simulink library "ddm"  (R2021b)
settings: Solver=VariableStepAuto  StartTime=0.0  StopTime=10.0  RelTol=1e-3
undefined symbols (not defined in the file or in its folder): ENUM_ADASACCSTA_ERROR, ENUM_ADASACCSTA_OFF, ENUM_ADASACCSTA_STANDBY, ENUM_ADASISASTA_OFF, ENUM_ALLOWMOV_ALLOWREADY, ENUM_APS, ENUM_BRKSTA_ERROR, ENUM_BRKSTA_OFF, ENUM_BRKSTA_ON, ENUM_BRKSW_INVALID, ENUM_BRKSW_OFF, ENUM_BRKSW_ON, ENUM_CHGPREACTERRSTA_OBCPRE, ENUM_DCDCFAULTSTA_ANYFAULTLV1, ENUM_DCDCFAULTSTA_ANYFAULTLV2, ENUM_DRIVETRAIN_AWD, ENUM_DRIVETRAIN_FWD, ENUM_DRIVETRAIN_RWD, ENUM_DRSEATSTA_INVALID, ENUM_EDUDRTSTA_NORMAL, ENUM_EPBSTA_APPLIED, ENUM_EPBSTA_RELEASED, ENUM_HVBATTREADYPRE_READY, ENUM_MCUWARN_LV0, ENUM_MCUWARN_LV1, ENUM_MCUWARN_LV2, ENUM_MCUWARN_LV3, ENUM_MCUWARN_NOERROR, ENUM_OBCFAULTSTA_ANYFAULT, ENUM_PAS_R2F2, ENUM_PDFAULT_BATTPDFAIL, ENUM_PDFAULT_DCDCDISABLE, ENUM_PDFAULT_MCUDISABLE, ENUM_PDFAULT_MCUDISCHRG, ENUM_POWERSTA_OFF, ENUM_POWERSTA_ON, ENUM_POWERSTA_READY, ENUM_POWERSTA_STANDBY, ENUM_PRESSINDI_LOW, ENUM_PUFAULT_BATTUPFAIL, ENUM_PUFAULT_DCDCENABLEFAIL, ENUM_PUFAULT_PRECHRGCHKFAIL, ENUM_PUFAULT_SAFETYCHKFAIL, ENUM_PUSTATE_COMPLETED, ENUM_PWRSTASW_OFF, ENUM_PWRSTASW_OFFA, ENUM_PWRSTASW_OFFCHVCHRG, ENUM_PWRSTASW_OFFCLVCHRG, ENUM_PWRSTASW_ON, ENUM_PWRSTASW_ONHVCHRG, ENUM_PWRSTASW_READY, ENUM_PWRSTASW_STANDBY, ENUM_RANGESTA_12IN, ENUM_SHIFTCOMMAND_D, ENUM_SHIFTCOMMAND_N, ENUM_SHIFTCOMMAND_P, ENUM_SHIFTCOMMAND_R, ENUM_VEHMALFUNLV_2ND, ENUM_VEHMALFUNLV_3RD, ENUM_VEHMALFUNLV_4TH ... (+835)
libraries: hcu_lib x750, $bdroot x12, simulink x5
(part 20 of 28)

== system ddm/DDM/DDM/PMM/SW failure/Hood switch failure ==
  note: Diagnostics and Fault Handling
  note: Fail Safe During Detection
  note: Fail Safe After Decision
  note: Release Condition After Decision
  note: Release Condition During Detection
  note: Test Pass Criteria
  note: Test Detection Criteria
  task_time_s : Inport
  VPMM_PowerSta_enum : Inport  Port=2
  VPMM_PwrStaSW_enum : Inport  Port=3
  VINP_HoodSW : Inport  Port=4
  DTC_clear_request : Inport  Port=5
  Constant{10,18,53,55} (4 alike) : Constant  Value=FALSE
  Constant11 : Constant  Value=KDDM_HoodSWPassTO_s
  Constant15 : Constant  Value=KDDM_HoodSWPassTO_s
  Constant16 : Constant  Value=KDDM_HoodSWDetTO_s
  Constant17 : Constant  Value=KDDM_HoodSW_s
  Constant19 : Constant  Value=ENUM_PWRSTASW_OFF
  Constant21 : Constant  Value=ZERO_INT
  Constant22 : Constant  Value=ENUM_PWRSTASW_OFF
  Constant{23,42,52,54} (4 alike) : Constant  Value=TRUE
  Constant24 : Constant  Value=KDDM_HoodSWPassTO_s
  Constant25 : Constant  Value=KDDM_HoodSWDTC_cnt
  Constant26 : Constant  Value=ONE_INT
  Constant32 : Constant  Value=ZERO_FLOAT
  Constant45 : Constant  Value=ENUM_POWERSTA_OFF
  Constant56 : Constant  Value=KDDM_HoodSWPassSW_flg
  Constant57 : Constant  Value=KDDM_HoodSWCFSSW_flg
  Constant58 : Constant  Value=KDDM_HoodSWDFSSW_flg
  Constant59 : Constant  Value=KDDM_HoodSWDetSW_flg
  Constant60 : Constant  Value=KDDM_HoodSWDTC_cnt
  DTC_Couter1 : hcu_lib/Basic_Blocks/DTC_Couter
  DTC_Info : hcu_lib/Basic_Blocks/DTC_Info
  Data Type Conversion12 : DataTypeConversion  OutDataTypeStr=boolean
  Data Type Conversion14 : DataTypeConversion  OutDataTypeStr=boolean
  Data Type Conversion4 : DataTypeConversion  OutDataTypeStr=uint8
  Data Type Conversion7 : DataTypeConversion
  Equal1 : RelationalOperator  Operator=~=  OutDataTypeStr=boolean  RndMeth=Simplest
  Equal3 : RelationalOperator  Operator=~=  OutDataTypeStr=boolean  RndMeth=Simplest
  Equal4 : RelationalOperator  Operator=~=  OutDataTypeStr=boolean  RndMeth=Simplest
  Equal5 : RelationalOperator  OutDataTypeStr=boolean  RndMeth=Simplest
  Equal8 : RelationalOperator  Operator===  OutDataTypeStr=boolean  RndMeth=Simplest
  Logical Operator{2,4..5,7} (4 alike) : Logic  Operator=NOT  AllPortsSameDT=off  OutDataTypeStr=boolean
  Logical Operator27 : Logic  Operator=OR  AllPortsSameDT=off  OutDataTypeStr=boolean
  Logical Operator{6,28..30} (4 alike) : Logic  AllPortsSameDT=off  OutDataTypeStr=boolean
  Logical Operator3 : Logic  Operator=OR  AllPortsSameDT=off  OutDataTypeStr=boolean
  Logical Operator31 : Logic  Inputs=3  AllPortsSameDT=off  OutDataTypeStr=boolean
  Logical Operator32 : Logic  Operator=OR  Inputs=3  AllPortsSameDT=off  OutDataTypeStr=boolean
  Logical Operator33 : Logic  Operator=OR  Inputs=3  AllPortsSameDT=off  OutDataTypeStr=boolean
  Relational Operator4 : RelationalOperator  Operator=<=  OutDataTypeStr=boolean  RndMeth=Simplest
  Relational Operator5 : RelationalOperator  Operator=>  OutDataTypeStr=boolean  RndMeth=Simplest
  Relay1 : Relay  OnSwitchValue=ONE_INT  OffSwitchValue=ZERO_INT
  SR_Latch1 : hcu_lib/Basic_Blocks/SR_Latch
  SR_Latch2 : hcu_lib/Basic_Blocks/SR_Latch
  SR_Latch3 : $bdroot/DDM/DDM/PMM/SW failure/Driver seat switch failure/SR_Latch3
  SR_Latch5 : hcu_lib/Basic_Blocks/SR_Latch
  Subsystem : $bdroot/DDM/DDM/PMM/SW failure/Driver seat switch failure/Subsystem  SystemSampleTime=-1  VariantActivationTime=update diagram  Latency=0  AutoFrameSizeCalculation=off
      link override Constant15: Value=KDDM_HoodSW_s
  Switch{5,10..11,14..16} (6 alike) : Switch  Criteria=u2 ~= 0
  Test Detection Criteria2 : hcu_lib/Basic_Blocks/Test Detection Criteria
  Timer : hcu_lib/Basic_Blocks/Test Detection Criteria/Timer
  Timer1 : hcu_lib/Basic_Blocks/Timer
  Unit Delay : UnitDelay  SampleTime=-1  HasFrameUpgradeWarning=on
  Unit Delay9 : UnitDelay  SampleTime=-1  HasFrameUpgradeWarning=on
  VDDM_HoodSWDTC_raw32 : Outport
  VDDM_VCUHoodSWSta_flg : Outport  Port=2
  wires:
  Logical Operator31/1 -> DTC_Couter1/1
  [DTC_clear_request] -> Logical Operator3/2
  SR_Latch5/1 -> Logical Operator30/1
  Logical Operator3/1 -> SR_Latch5/2
  Logical Operator28/1 -> [VDDM_HoodSWDFS_flg]
  Logical Operator2/1 -> Logical Operator31/3
  [VDDM_HoodSWPass_flg] -> Logical Operator33/1
  DTC_Couter1/2 -> Data Type Conversion4/1
  [DTC_clear_request] -> Logical Operator2/1
  [DTC_clear_request] -> Logical Operator32/3
  [DTC_clear_request] -> Logical Operator33/3
  Logical Operator33/1 -> Logical Operator29/1
  Data Type Conversion4/1 -> [VDDM_HoodSWDTC_cnt]  "VDDM_HoodSWDTC_cnt"
  Relay1/1 -> SR_Latch2/1
  [VDDM_HoodSWCFSRls_flg] -> Logical Operator3/1
  [VDDM_HoodSWDTC_cnt] -> Relay1/1
  [VDDM_HoodSWDet_flg] -> Logical Operator31/1
  Constant57/1 -> Logical Operator30/2
  Logical Operator32/1 -> SR_Latch2/2
  Logical Operator29/1 -> DTC_Couter1/2
  Logical Operator30/1 -> [VDDM_HoodSWCFS_flg]  "VDDM_HoodSWCFS_flg"
  Constant58/1 -> Logical Operator28/1
  Constant59/1 -> Logical Operator31/2
  Constant60/1 -> DTC_Couter1/3
  Constant56/1 -> Logical Operator29/2
  [VDDM_HoodSWDFSRls_flg] -> Logical Operator32/1
  DTC_Couter1/1 -> SR_Latch5/1
  [VDDM_HoodSWCFSRls_flg] -> Logical Operator33/2
  [VDDM_HoodSWCFS_flg] -> Logical Operator32/2
  SR_Latch2/1 -> Logical Operator28/2
  [DTC_clear_request] -> DTC_Info/4
  [VDDM_HoodSWDet_flg] -> DTC_Info/1
  [VDDM_HoodSWCFS_flg] -> DTC_Info/3
  [VDDM_HoodSWPass_flg] -> DTC_Info/2
  DTC_Info/1 -> VDDM_HoodSWDTC_raw32/1  "VDDM_HoodSWDTC_raw32"
  Constant10/1 -> Switch11/3
  VPMM_PwrStaSW_enum/1 -> [VPMM_PwrStaSW_enum]
  VPMM_PowerSta_enum/1 -> [VPMM_PowerSta_enum]
  DTC_clear_request/1 -> [DTC_clear_request]
  VINP_HoodSW/1 -> [VINP_HoodSWGPIO_flg]
  task_time_s/1 -> [task_time_s]
  [VDDM_HoodSWCFS_flg] -> Switch11/2
  Constant42/1 -> Switch11/1
  Switch11/1 -> [VDDM_VCUHoodSWSta_flg]  "VDDM_VCUHoodSWSta_flg"
  Logical Operator27/1 -> Switch15/2
  Constant52/1 -> Switch16/1
  Equal8/1 -> Logical Operator27/1
  [VDDM_HoodSWPass_flg] -> Switch16/2
  Constant53/1 -> Switch16/3
  Constant45/1 -> Equal8/2
  Constant55/1 -> Switch15/3
  Switch15/1 -> [VDDM_HoodSWCFSRls_flg]  "VDDM_HoodSWCFSRls_flg"
  Switch16/1 -> [VDDM_HoodSWDFSRls_flg]
  [DTC_clear_request] -> Logical Operator27/2
  Constant54/1 -> Switch15/1
  [VPMM_PowerSta_enum] -> Equal8/1
  [VDDM_VCUHoodSWSta_flg] -> VDDM_VCUHoodSWSta_flg/1
  [VDDM_HoodSWChange_flg] -> SR_Latch1/2
  Logical Operator7/1 -> Timer1/1
  Data Type Conversion7/1 -> Test Detection Criteria2/4
  Subsystem/1 -> Logical Operator6/1
  Equal4/1 -> [VDDM_HoodSWChange_flg]
  Test Detection Criteria2/1 -> [VDDM_HoodSWDet_flg]  "VDDM_HoodSWDet_flg"
  Switch10/1 -> Logical Operator7/1, Timer1/2
  Constant32/1 -> Relational Operator5/2
  [VPMM_PwrStaSW_enum] -> Equal1/1
  [VDDM_xxx_flg] -> SR_Latch3/2
  Relational Operator4/1 -> Logical Operator6/2
  Constant26/1 -> SR_Latch1/1
  [task_time_s] -> Timer1/3
  Constant21/1 -> Switch14/3
  [task_time_s] -> Timer/3
  Constant22/1 -> Equal1/2
  Data Type Conversion14/1 -> Equal4/1
  SR_Latch1/1 -> Logical Operator5/1, Logical Operator4/1, Timer/1
  Switch5/1 -> Data Type Conversion12/1
  Constant23/1 -> Switch10/3
  Data Type Conversion12/1 -> Test Detection Criteria2/1
  Logical Operator6/1 -> [HoodSWFault_flg], Switch14/1
  Constant17/1 -> Relational Operator4/2
  Constant11/1 -> Timer/4
  Unit Delay/1 -> Subsystem/1
  Logical Operator4/1 -> Timer/2
  Constant25/1 -> Test Detection Criteria2/3
  [task_time_s] -> Test Detection Criteria2/2
  Constant18/1 -> Switch5/1
  Relational Operator5/1 -> Unit Delay9/1, Equal4/2
  [DTC_clear_request] -> Switch5/2
  Logical Operator5/1 -> Subsystem/Trigger
  Constant16/1 -> Data Type Conversion7/1
  Constant24/1 -> Equal5/2
  Timer1/1 -> Equal5/1
  Timer/1 -> Relational Operator4/1, Unit Delay/1
  Constant15/1 -> Timer1/4
  Unit Delay9/1 -> Data Type Conversion14/1
  Equal3/1 -> Switch10/2
  Equal5/1 -> SR_Latch3/1
  Equal1/1 -> Switch14/2
  Switch14/1 -> [VDDM_xxx_flg], Switch5/3
  [HoodSWFault_flg] -> Switch10/1
  [VINP_HoodSWGPIO_flg] -> Relational Operator5/1
  [VPMM_PwrStaSW_enum] -> Equal3/1
  SR_Latch3/1 -> [VDDM_HoodSWPass_flg]  "VDDM_HoodSWPass_flg"
  Constant19/1 -> Equal3/2

== system ddm/DDM/DDM/PMM/SW failure/RL Door switch failure ==
  note: Diagnostics and Fault Handling
  note: Release Condition During Detection
  note: Release Condition After Decision
  note: Fail Safe After Decision
  note: Fail Safe During Detection
  note: Test Pass Criteria
  note: Test Detection Criteria
  task_time_s : Inport
  VPMM_PowerSta_enum : Inport  Port=2
  VPMM_PwrStaSW_enum : Inport  Port=3
  VINP_RLAJARSW : Inport  Port=4
  DTC_clear_request : Inport  Port=5
  Constant{10,18,53,55} (4 alike) : Constant  Value=FALSE
  Constant11 : Constant  Value=KDDM_RLDoorSWPassTO_s
  Constant15 : Constant  Value=KDDM_RLDoorSWPassTO_s
  Constant16 : Constant  Value=KDDM_RLDoorSWDetTO_s
  Constant17 : Constant  Value=KDDM_RLDoorSW_s
  Constant19 : Constant  Value=ENUM_PWRSTASW_OFF
  Constant21 : Constant  Value=ZERO_INT
  Constant22 : Constant  Value=ENUM_PWRSTASW_OFF
  Constant{23,42,52,54} (4 alike) : Constant  Value=TRUE
  Constant24 : Constant  Value=KDDM_RLDoorSWPassTO_s
  Constant25 : Constant  Value=KDDM_RLDoorSWDTC_cnt
  Constant26 : Constant  Value=ONE_INT
  Constant32 : Constant  Value=ZERO_FLOAT
  Constant45 : Constant  Value=ENUM_POWERSTA_OFF
  Constant56 : Constant  Value=KDDM_RLDoorSWPassSW_flg
  Constant57 : Constant  Value=KDDM_RLDoorSWCFSSW_flg
  Constant58 : Constant  Value=KDDM_RLDoorSWDFSSW_flg
  Constant59 : Constant  Value=KDDM_RLDoorSWDetSW_flg
  Constant60 : Constant  Value=KDDM_RLDoorSWDTC_cnt
  DTC_Couter1 : hcu_lib/Basic_Blocks/DTC_Couter
  DTC_Info : hcu_lib/Basic_Blocks/DTC_Info
  Data Type Conversion10 : DataTypeConversion  OutDataTypeStr=boolean
  Data Type Conversion13 : DataTypeConversion
  Data Type Conversion14 : DataTypeConversion  OutDataTypeStr=boolean
  Data Type Conversion4 : DataTypeConversion  OutDataTypeStr=uint8
  Equal1 : RelationalOperator  Operator=~=  OutDataTypeStr=boolean  RndMeth=Simplest
  Equal3 : RelationalOperator  Operator=~=  OutDataTypeStr=boolean  RndMeth=Simplest
  Equal4 : RelationalOperator  Operator=~=  OutDataTypeStr=boolean  RndMeth=Simplest
  Equal5 : RelationalOperator  OutDataTypeStr=boolean  RndMeth=Simplest
  Equal8 : RelationalOperator  Operator===  OutDataTypeStr=boolean  RndMeth=Simplest
  Logical Operator{2,4..5,7} (4 alike) : Logic  Operator=NOT  AllPortsSameDT=off  OutDataTypeStr=boolean
  Logical Operator27 : Logic  Operator=OR  AllPortsSameDT=off  OutDataTypeStr=boolean
  Logical Operator{6,28..30} (4 alike) : Logic  AllPortsSameDT=off  OutDataTypeStr=boolean
  Logical Operator3 : Logic  Operator=OR  AllPortsSameDT=off  OutDataTypeStr=boolean
  Logical Operator31 : Logic  Inputs=3  AllPortsSameDT=off  OutDataTypeStr=boolean
  Logical Operator32 : Logic  Operator=OR  Inputs=3  AllPortsSameDT=off  OutDataTypeStr=boolean
  Logical Operator33 : Logic  Operator=OR  Inputs=3  AllPortsSameDT=off  OutDataTypeStr=boolean
  Relational Operator4 : RelationalOperator  Operator=<=  OutDataTypeStr=boolean  RndMeth=Simplest
  Relational Operator5 : RelationalOperator  Operator=>  OutDataTypeStr=boolean  RndMeth=Simplest
  Relay1 : Relay  OnSwitchValue=ONE_INT  OffSwitchValue=ZERO_INT
  SR_Latch1 : hcu_lib/Basic_Blocks/SR_Latch
  SR_Latch2 : hcu_lib/Basic_Blocks/SR_Latch
  SR_Latch3 : $bdroot/DDM/DDM/PMM/SW failure/Driver seat switch failure/SR_Latch3
  SR_Latch5 : hcu_lib/Basic_Blocks/SR_Latch
  Subsystem : $bdroot/DDM/DDM/PMM/SW failure/Driver seat switch failure/Subsystem  SystemSampleTime=-1  VariantActivationTime=update diagram  Latency=0  AutoFrameSizeCalculation=off
      link override Constant15: Value=KDDM_RLDoorSW_s
  Switch{5,10..11,14..16} (6 alike) : Switch  Criteria=u2 ~= 0
  Test Detection Criteria2 : hcu_lib/Basic_Blocks/Test Detection Criteria
  Timer : hcu_lib/Basic_Blocks/Test Detection Criteria/Timer
  Timer1 : hcu_lib/Basic_Blocks/Timer
  Unit Delay : UnitDelay  SampleTime=-1  HasFrameUpgradeWarning=on
  Unit Delay9 : UnitDelay  SampleTime=-1  HasFrameUpgradeWarning=on
  VDDM_RLDoorSWDTC_raw32 : Outport
  VDDM_VCURLDoorSta_flg : Outport  Port=2
  wires:
  Data Type Conversion4/1 -> [VDDM_RLDoorSWDTC_cnt]
  [VDDM_RLDoorSWPass_flg] -> Logical Operator33/1
  DTC_Couter1/1 -> SR_Latch5/1
  SR_Latch2/1 -> Logical Operator28/2
  [DTC_clear_request] -> Logical Operator32/3
  [VDDM_RLDoorSWCFSRls_flg] -> Logical Operator3/1
  Logical Operator2/1 -> Logical Operator31/3
  [VDDM_RLDoorSWCFSRls_flg] -> Logical Operator33/2
  Logical Operator30/1 -> [VDDM_RLDoorSWCFS_flg]  "VDDM_RLDoorSWCFS_flg"
  Constant56/1 -> Logical Operator29/2
  Constant57/1 -> Logical Operator30/2
  Constant59/1 -> Logical Operator31/2
  Logical Operator29/1 -> DTC_Couter1/2
  DTC_Couter1/2 -> Data Type Conversion4/1
  SR_Latch5/1 -> Logical Operator30/1
  [VDDM_RLDoorSWDFSRls_flg] -> Logical Operator32/1
  [VDDM_RLDoorSWDTC_cnt] -> Relay1/1
  [VDDM_RLDoorSWDet_flg] -> Logical Operator31/1
  Logical Operator3/1 -> SR_Latch5/2
  Relay1/1 -> SR_Latch2/1
  Constant58/1 -> Logical Operator28/1
  Logical Operator32/1 -> SR_Latch2/2
  Logical Operator28/1 -> [VDDM_RLDoorSWDFS_flg]
  [DTC_clear_request] -> Logical Operator3/2
  [DTC_clear_request] -> Logical Operator33/3
  [VDDM_RLDoorSWCFS_flg] -> Logical Operator32/2
  Logical Operator33/1 -> Logical Operator29/1
  Logical Operator31/1 -> DTC_Couter1/1
  [DTC_clear_request] -> Logical Operator2/1
  Constant60/1 -> DTC_Couter1/3
  [DTC_clear_request] -> DTC_Info/4
  [VDDM_RLDoorSWDet_flg] -> DTC_Info/1
  DTC_Info/1 -> VDDM_RLDoorSWDTC_raw32/1  "VDDM_RLDoorSWDTC_raw32"
  [VDDM_RLDoorSWCFS_flg] -> DTC_Info/3
  [VDDM_RLDoorSWPass_flg] -> DTC_Info/2
  Constant10/1 -> Switch11/3
  VPMM_PowerSta_enum/1 -> [VPMM_PowerSta_enum]
  VPMM_PwrStaSW_enum/1 -> [VPMM_PwrStaSW_enum]
  [VDDM_VCURLDoorSta_flg] -> VDDM_VCURLDoorSta_flg/1
  [VPMM_PowerSta_enum] -> Equal8/1
  Constant54/1 -> Switch15/1
  [DTC_clear_request] -> Logical Operator27/2
  Switch16/1 -> [VDDM_RLDoorSWDFSRls_flg]
  Switch15/1 -> [VDDM_RLDoorSWCFSRls_flg]  "VDDM_RLDoorSWCFSRls_flg"
  Constant55/1 -> Switch15/3
  Constant45/1 -> Equal8/2
  Constant53/1 -> Switch16/3
  [VDDM_RLDoorSWPass_flg] -> Switch16/2
  Equal8/1 -> Logical Operator27/1
  Constant52/1 -> Switch16/1
  Logical Operator27/1 -> Switch15/2
  Switch11/1 -> [VDDM_VCURLDoorSta_flg]  "VDDM_VCURLDoorSta_flg"
  Constant42/1 -> Switch11/1
  [VDDM_RLDoorSWCFS_flg] -> Switch11/2
  task_time_s/1 -> [task_time_s]
  VINP_RLAJARSW/1 -> [VINP_RL_AJAR_SW]
  DTC_clear_request/1 -> [DTC_clear_request]
  Data Type Conversion14/1 -> Equal4/1
  Constant23/1 -> Switch10/3
  [task_time_s] -> Timer1/3
  Constant22/1 -> Equal1/2
  [task_time_s] -> Timer/3
  Constant21/1 -> Switch14/3
  Constant26/1 -> SR_Latch1/1
  [task_time_s] -> Test Detection Criteria2/2
  [RLDoorSWFault_flg] -> Switch10/1
  Logical Operator7/1 -> Timer1/1
  Timer1/1 -> Equal5/1
  Logical Operator4/1 -> Timer/2
  Data Type Conversion10/1 -> Test Detection Criteria2/1
  Data Type Conversion13/1 -> Test Detection Criteria2/4
  [VDDM_xxx_flg] -> SR_Latch3/2
  Unit Delay/1 -> Subsystem/1
  Constant25/1 -> Test Detection Criteria2/3
  Constant24/1 -> Equal5/2
  Subsystem/1 -> Logical Operator6/1
  Equal1/1 -> Switch14/2
  [DTC_clear_request] -> Switch5/2
  Constant16/1 -> Data Type Conversion13/1
  [VPMM_PwrStaSW_enum] -> Equal3/1
  Constant11/1 -> Timer/4
  Switch5/1 -> Data Type Conversion10/1
  Switch14/1 -> [VDDM_xxx_flg], Switch5/3
  SR_Latch1/1 -> Logical Operator5/1, Logical Operator4/1, Timer/1
  Relational Operator4/1 -> Logical Operator6/2
  Constant18/1 -> Switch5/1
  SR_Latch3/1 -> [VDDM_RLDoorSWPass_flg]  "VDDM_RLDoorSWPass_flg"
  Equal5/1 -> SR_Latch3/1
  Constant17/1 -> Relational Operator4/2
  Constant15/1 -> Timer1/4
  Equal3/1 -> Switch10/2
  Logical Operator6/1 -> [RLDoorSWFault_flg], Switch14/1
  [VPMM_PwrStaSW_enum] -> Equal1/1
  Logical Operator5/1 -> Subsystem/Trigger
  [VDDM_RLDoorSWChange_flg] -> SR_Latch1/2
  Relational Operator5/1 -> Unit Delay9/1, Equal4/2
  Unit Delay9/1 -> Data Type Conversion14/1
  Timer/1 -> Relational Operator4/1, Unit Delay/1
  [VINP_RL_AJAR_SW] -> Relational Operator5/1
  Constant19/1 -> Equal3/2
  Equal4/1 -> [VDDM_RLDoorSWChange_flg]
  Switch10/1 -> Logical Operator7/1, Timer1/2
  Constant32/1 -> Relational Operator5/2
  Test Detection Criteria2/1 -> [VDDM_RLDoorSWDet_flg]  "VDDM_RLDoorSWDet_flg"

== system ddm/DDM/DDM/PMM/SW failure/RR Door switch failure ==
  note: Diagnostics and Fault Handling
  note: Fail Safe During Detection
  note: Fail Safe After Decision
  note: Release Condition After Decision
  note: Release Condition During Detection
  note: Test Detection Criteria
  note: Test Pass Criteria
  task_time_s : Inport
  VPMM_PowerSta_enum : Inport  Port=2
  VPMM_PwrStaSW_enum : Inport  Port=3
  VINP_RRAJARSW : Inport  Port=4
  DTC_clear_request : Inport  Port=5
  Constant{10,18,53,55} (4 alike) : Constant  Value=FALSE
  Constant11 : Constant  Value=KDDM_RRDoorSWPassTO_s
  Constant15 : Constant  Value=KDDM_RRDoorSWPassTO_s
  Constant16 : Constant  Value=KDDM_RRDoorSWDetTO_s
  Constant17 : Constant  Value=KDDM_RRDoorSW_s
  Constant19 : Constant  Value=ENUM_PWRSTASW_OFF
  Constant21 : Constant  Value=ZERO_INT
  Constant22 : Constant  Value=ENUM_PWRSTASW_OFF
  Constant{23,42,52,54} (4 alike) : Constant  Value=TRUE
  Constant24 : Constant  Value=KDDM_RRDoorSWPassTO_s
  Constant25 : Constant  Value=KDDM_RRDoorSWDTC_cnt
  Constant26 : Constant  Value=ONE_INT
  Constant32 : Constant  Value=ZERO_FLOAT
  Constant45 : Constant  Value=ENUM_POWERSTA_OFF
  Constant56 : Constant  Value=KDDM_RRDoorSWPassSW_flg
  Constant57 : Constant  Value=KDDM_RRDoorSWCFSSW_flg
  Constant58 : Constant  Value=KDDM_RRDoorSWDFSSW_flg
  Constant59 : Constant  Value=KDDM_RRDoorSWDetSW_flg
  Constant60 : Constant  Value=KDDM_RRDoorSWDTC_cnt
  DTC_Couter1 : hcu_lib/Basic_Blocks/DTC_Couter
  DTC_Info : hcu_lib/Basic_Blocks/DTC_Info
  Data Type Conversion12 : DataTypeConversion  OutDataTypeStr=boolean
  Data Type Conversion14 : DataTypeConversion  OutDataTypeStr=boolean
  Data Type Conversion4 : DataTypeConversion  OutDataTypeStr=uint8
  Data Type Conversion7 : DataTypeConversion
  Equal1 : RelationalOperator  Operator=~=  OutDataTypeStr=boolean  RndMeth=Simplest
  Equal3 : RelationalOperator  Operator=~=  OutDataTypeStr=boolean  RndMeth=Simplest
  Equal4 : RelationalOperator  Operator=~=  OutDataTypeStr=boolean  RndMeth=Simplest
  Equal5 : RelationalOperator  OutDataTypeStr=boolean  RndMeth=Simplest
  Equal8 : RelationalOperator  Operator===  OutDataTypeStr=boolean  RndMeth=Simplest
  Logical Operator{2,4..5,7} (4 alike) : Logic  Operator=NOT  AllPortsSameDT=off  OutDataTypeStr=boolean
  Logical Operator27 : Logic  Operator=OR  AllPortsSameDT=off  OutDataTypeStr=boolean
  Logical Operator{6,28..30} (4 alike) : Logic  AllPortsSameDT=off  OutDataTypeStr=boolean
  Logical Operator3 : Logic  Operator=OR  AllPortsSameDT=off  OutDataTypeStr=boolean
  Logical Operator31 : Logic  Inputs=3  AllPortsSameDT=off  OutDataTypeStr=boolean
  Logical Operator32 : Logic  Operator=OR  Inputs=3  AllPortsSameDT=off  OutDataTypeStr=boolean
  Logical Operator33 : Logic  Operator=OR  Inputs=3  AllPortsSameDT=off  OutDataTypeStr=boolean
  Relational Operator4 : RelationalOperator  Operator=<=  OutDataTypeStr=boolean  RndMeth=Simplest
  Relational Operator5 : RelationalOperator  Operator=>  OutDataTypeStr=boolean  RndMeth=Simplest
  Relay1 : Relay  OnSwitchValue=ONE_INT  OffSwitchValue=ZERO_INT
  SR_Latch1 : hcu_lib/Basic_Blocks/SR_Latch
  SR_Latch2 : hcu_lib/Basic_Blocks/SR_Latch
  SR_Latch3 : $bdroot/DDM/DDM/PMM/SW failure/Driver seat switch failure/SR_Latch3
  SR_Latch5 : hcu_lib/Basic_Blocks/SR_Latch
  Subsystem : $bdroot/DDM/DDM/PMM/SW failure/Driver seat switch failure/Subsystem  SystemSampleTime=-1  VariantActivationTime=update diagram  Latency=0  AutoFrameSizeCalculation=off
      link override Constant15: Value=KDDM_RRDoorSW_s
  Switch{5,10..11,14..16} (6 alike) : Switch  Criteria=u2 ~= 0
  Test Detection Criteria2 : hcu_lib/Basic_Blocks/Test Detection Criteria
  Timer : hcu_lib/Basic_Blocks/Test Detection Criteria/Timer
  Timer1 : hcu_lib/Basic_Blocks/Timer
  Unit Delay : UnitDelay  SampleTime=-1  HasFrameUpgradeWarning=on
  Unit Delay9 : UnitDelay  SampleTime=-1  HasFrameUpgradeWarning=on
  VDDM_RRDoorSWDTC_raw32 : Outport
  VDDM_VCURRDoorSta_flg : Outport  Port=2
  wires:
  [DTC_clear_request] -> Logical Operator33/3
  [VDDM_RRDoorSWPass_flg] -> Logical Operator33/1
  [DTC_clear_request] -> Logical Operator32/3
  [VDDM_RRDoorSWDTC_cnt] -> Relay1/1
  [DTC_clear_request] -> Logical Operator2/1
  [DTC_clear_request] -> Logical Operator3/2
  [VDDM_RRDoorSWDet_flg] -> Logical Operator31/1
  Logical Operator2/1 -> Logical Operator31/3
  Constant57/1 -> Logical Operator30/2
  Logical Operator29/1 -> DTC_Couter1/2
  [VDDM_RRDoorSWDFSRls_flg] -> Logical Operator32/1
  DTC_Couter1/2 -> Data Type Conversion4/1
  Constant56/1 -> Logical Operator29/2
  Data Type Conversion4/1 -> [VDDM_RRDoorSWDTC_cnt]  "VDDM_RRDoorSWDTC_cnt"
  [VDDM_RRDoorSWCFSRls_flg] -> Logical Operator3/1
  Logical Operator31/1 -> DTC_Couter1/1
  Relay1/1 -> SR_Latch2/1
  DTC_Couter1/1 -> SR_Latch5/1
  SR_Latch2/1 -> Logical Operator28/2
  Logical Operator28/1 -> [VDDM_RRDoorSWDFS_flg]
  Logical Operator3/1 -> SR_Latch5/2
  Logical Operator32/1 -> SR_Latch2/2
  Constant60/1 -> DTC_Couter1/3
  Constant58/1 -> Logical Operator28/1
  [VDDM_RRDoorSWCFSRls_flg] -> Logical Operator33/2
  Logical Operator30/1 -> [VDDM_RRDoorSWCFS_flg]  "VDDM_RRDoorSWCFS_flg"
  Logical Operator33/1 -> Logical Operator29/1
  SR_Latch5/1 -> Logical Operator30/1
  Constant59/1 -> Logical Operator31/2
  [VDDM_RRDoorSWCFS_flg] -> Logical Operator32/2
  [DTC_clear_request] -> DTC_Info/4
  [VDDM_RRDoorSWDet_flg] -> DTC_Info/1
  [VDDM_RRDoorSWCFS_flg] -> DTC_Info/3
  [VDDM_RRDoorSWPass_flg] -> DTC_Info/2
  DTC_Info/1 -> VDDM_RRDoorSWDTC_raw32/1  "VDDM_RRDoorSWDTC_raw32"
  Constant10/1 -> Switch11/3
  VPMM_PwrStaSW_enum/1 -> [VPMM_PwrStaSW_enum]
  VPMM_PowerSta_enum/1 -> [VPMM_PowerSta_enum]
  DTC_clear_request/1 -> [DTC_clear_request]
  VINP_RRAJARSW/1 -> [VINP_RR_AJAR_SW]
  task_time_s/1 -> [task_time_s]
  [VDDM_RRDoorSWCFS_flg] -> Switch11/2
  Constant42/1 -> Switch11/1
  Switch11/1 -> [VDDM_VCURRDoorSta_flg]  "VDDM_VCURRDoorSta_flg"
  Logical Operator27/1 -> Switch15/2
  Constant52/1 -> Switch16/1
  Equal8/1 -> Logical Operator27/1
  [VDDM_RRDoorSWPass_flg] -> Switch16/2
  Constant53/1 -> Switch16/3
  Constant45/1 -> Equal8/2
  Constant55/1 -> Switch15/3
  Switch15/1 -> [VDDM_RRDoorSWCFSRls_flg]  "VDDM_RRDoorSWCFSRls_flg"
  Switch16/1 -> [VDDM_RRDoorSWDFSRls_flg]
  [DTC_clear_request] -> Logical Operator27/2
  Constant54/1 -> Switch15/1
  [VPMM_PowerSta_enum] -> Equal8/1
  [VDDM_VCURRDoorSta_flg] -> VDDM_VCURRDoorSta_flg/1
  Equal5/1 -> SR_Latch3/1
  Equal3/1 -> Switch10/2
  Constant15/1 -> Timer1/4
  SR_Latch3/1 -> [VDDM_RRDoorSWPass_flg]  "VDDM_RRDoorSWPass_flg"
  [VDDM_RRDoorSWChange_flg] -> SR_Latch1/2
  Switch14/1 -> [VDDM_xxx_flg], Switch5/3
  Switch5/1 -> Data Type Conversion12/1
  Logical Operator6/1 -> [RRDoorSWFault_flg], Switch14/1
  [VPMM_PwrStaSW_enum] -> Equal3/1
  Constant11/1 -> Timer/4
  Logical Operator4/1 -> Timer/2
  Data Type Conversion12/1 -> Test Detection Criteria2/1
  Unit Delay/1 -> Subsystem/1
  Constant21/1 -> Switch14/3
  [task_time_s] -> Timer/3
  [task_time_s] -> Timer1/3
  Constant26/1 -> SR_Latch1/1
  Constant22/1 -> Equal1/2
  Data Type Conversion14/1 -> Equal4/1
  SR_Latch1/1 -> Logical Operator5/1, Logical Operator4/1, Timer/1
  Constant23/1 -> Switch10/3
  [VDDM_xxx_flg] -> SR_Latch3/2
  [VINP_RR_AJAR_SW] -> Relational Operator5/1
  Relational Operator4/1 -> Logical Operator6/2
  [VPMM_PwrStaSW_enum] -> Equal1/1
  Logical Operator5/1 -> Subsystem/Trigger
  Test Detection Criteria2/1 -> [VDDM_RRDoorSWDet_flg]  "VDDM_RRDoorSWDet_flg"
  Constant17/1 -> Relational Operator4/2
  Constant32/1 -> Relational Operator5/2
  Constant16/1 -> Data Type Conversion7/1
  Switch10/1 -> Logical Operator7/1, Timer1/2
  Subsystem/1 -> Logical Operator6/1
  Equal4/1 -> [VDDM_RRDoorSWChange_flg]
  [task_time_s] -> Test Detection Criteria2/2
  Equal1/1 -> Switch14/2
  Logical Operator7/1 -> Timer1/1
  Unit Delay9/1 -> Data Type Conversion14/1
  Data Type Conversion7/1 -> Test Detection Criteria2/4
  Timer1/1 -> Equal5/1
  Constant19/1 -> Equal3/2
  Constant24/1 -> Equal5/2
  Timer/1 -> Relational Operator4/1, Unit Delay/1
  [DTC_clear_request] -> Switch5/2
  Relational Operator5/1 -> Unit Delay9/1, Equal4/2
  Constant25/1 -> Test Detection Criteria2/3
  [RRDoorSWFault_flg] -> Switch10/1
  Constant18/1 -> Switch5/1

== system ddm/DDM/DDM/PMM/SW failure/Tailgate switch failure ==
  note: Diagnostics and Fault Handling
  note: Release Condition During Detection
  note: Release Condition After Decision
  note: Fail Safe After Decision
  note: Fail Safe During Detection
  note: Test Pass Criteria
  note: Test Detection Criteria
  task_time_s : Inport
  VPMM_PowerSta_enum : Inport  Port=2
  VPMM_PwrStaSW_enum : Inport  Port=3
  VINP_TailgaSW : Inport  Port=4
  DTC_clear_request : Inport  Port=5
  Constant{10,18,53,55} (4 alike) : Constant  Value=FALSE
  Constant11 : Constant  Value=KDDM_TailgaSWPassTO_s
  Constant15 : Constant  Value=KDDM_TailgaSWPassTO_s
  Constant16 : Constant  Value=KDDM_TailgaSWDetTO_s
  Constant17 : Constant  Value=KDDM_TailgaSW_s
  Constant19 : Constant  Value=ENUM_PWRSTASW_OFF
  Constant21 : Constant  Value=ZERO_INT
  Constant22 : Constant  Value=ENUM_PWRSTASW_OFF
  Constant{23,42,52,54} (4 alike) : Constant  Value=TRUE
  Constant24 : Constant  Value=KDDM_TailgaSWPassTO_s
  Constant25 : Constant  Value=KDDM_TailgaSWDTC_cnt
  Constant26 : Constant  Value=ONE_INT
  Constant32 : Constant  Value=ZERO_FLOAT
  Constant45 : Constant  Value=ENUM_POWERSTA_OFF
  Constant56 : Constant  Value=KDDM_TailgaSWPassSW_flg
  Constant57 : Constant  Value=KDDM_TailgaSWCFSSW_flg
  Constant58 : Constant  Value=KDDM_TailgaSWDFSSW_flg
  Constant59 : Constant  Value=KDDM_TailgaSWDetSW_flg
  Constant60 : Constant  Value=KDDM_TailgaSWDTC_cnt
  DTC_Couter1 : hcu_lib/Basic_Blocks/DTC_Couter
  DTC_Info : hcu_lib/Basic_Blocks/DTC_Info
  Data Type Conversion12 : DataTypeConversion  OutDataTypeStr=boolean
  Data Type Conversion14 : DataTypeConversion  OutDataTypeStr=boolean
  Data Type Conversion4 : DataTypeConversion  OutDataTypeStr=uint8
  Data Type Conversion7 : DataTypeConversion
  Equal1 : RelationalOperator  Operator=~=  OutDataTypeStr=boolean  RndMeth=Simplest
  Equal3 : RelationalOperator  Operator=~=  OutDataTypeStr=boolean  RndMeth=Simplest
  Equal4 : RelationalOperator  Operator=~=  OutDataTypeStr=boolean  RndMeth=Simplest
  Equal5 : RelationalOperator  OutDataTypeStr=boolean  RndMeth=Simplest
  Equal8 : RelationalOperator  Operator===  OutDataTypeStr=boolean  RndMeth=Simplest
  Logical Operator{2,4..5,7} (4 alike) : Logic  Operator=NOT  AllPortsSameDT=off  OutDataTypeStr=boolean
  Logical Operator27 : Logic  Operator=OR  AllPortsSameDT=off  OutDataTypeStr=boolean
  Logical Operator{6,28..30} (4 alike) : Logic  AllPortsSameDT=off  OutDataTypeStr=boolean
  Logical Operator3 : Logic  Operator=OR  AllPortsSameDT=off  OutDataTypeStr=boolean
  Logical Operator31 : Logic  Inputs=3  AllPortsSameDT=off  OutDataTypeStr=boolean
  Logical Operator32 : Logic  Operator=OR  Inputs=3  AllPortsSameDT=off  OutDataTypeStr=boolean
  Logical Operator33 : Logic  Operator=OR  Inputs=3  AllPortsSameDT=off  OutDataTypeStr=boolean
  Relational Operator4 : RelationalOperator  Operator=<=  OutDataTypeStr=boolean  RndMeth=Simplest
  Relational Operator5 : RelationalOperator  Operator=>  OutDataTypeStr=boolean  RndMeth=Simplest
  Relay1 : Relay  OnSwitchValue=ONE_INT  OffSwitchValue=ZERO_INT
  SR_Latch1 : hcu_lib/Basic_Blocks/SR_Latch
  SR_Latch2 : hcu_lib/Basic_Blocks/SR_Latch
  SR_Latch3 : $bdroot/DDM/DDM/PMM/SW failure/Driver seat switch failure/SR_Latch3
  SR_Latch5 : hcu_lib/Basic_Blocks/SR_Latch
  Subsystem : $bdroot/DDM/DDM/PMM/SW failure/Driver seat switch failure/Subsystem  SystemSampleTime=-1  VariantActivationTime=update diagram  Latency=0  AutoFrameSizeCalculation=off
      link override Constant15: Value=KDDM_TailgaSW_s
  Switch{5,10..11,14..16} (6 alike) : Switch  Criteria=u2 ~= 0
  Test Detection Criteria2 : hcu_lib/Basic_Blocks/Test Detection Criteria
  Timer : hcu_lib/Basic_Blocks/Test Detection Criteria/Timer
  Timer1 : hcu_lib/Basic_Blocks/Timer
  Unit Delay : UnitDelay  SampleTime=-1  HasFrameUpgradeWarning=on
  Unit Delay9 : UnitDelay  SampleTime=-1  HasFrameUpgradeWarning=on
  VDDM_TailgaSWDTC_raw32 : Outport
  VDDM_VCUTailgateSWSta_flg : Outport  Port=2
  wires:
  Constant58/1 -> Logical Operator28/1
  [DTC_clear_request] -> Logical Operator32/3
  [DTC_clear_request] -> Logical Operator3/2
  [VDDM_TailgaSWPass_flg] -> Logical Operator33/1
  [DTC_clear_request] -> Logical Operator2/1
  Logical Operator3/1 -> SR_Latch5/2
  Logical Operator2/1 -> Logical Operator31/3
  Constant57/1 -> Logical Operator30/2
  [DTC_clear_request] -> Logical Operator33/3
  Logical Operator28/1 -> [VDDM_TailgaSWDFS_flg]
  Logical Operator30/1 -> [VDDM_TailgaSWCFS_flg]  "VDDM_TailgaSWCFS_flg"
  [VDDM_TailgaSWCFSRls_flg] -> Logical Operator33/2
  SR_Latch5/1 -> Logical Operator30/1
  Logical Operator33/1 -> Logical Operator29/1
  DTC_Couter1/1 -> SR_Latch5/1
  Logical Operator31/1 -> DTC_Couter1/1
  [VDDM_TailgaSWCFS_flg] -> Logical Operator32/2
  Data Type Conversion4/1 -> [VDDM_TailgaSWDTC_cnt]  "VDDM_TailgaSWDTC_cnt"
  [VDDM_TailgaSWDTC_cnt] -> Relay1/1
  DTC_Couter1/2 -> Data Type Conversion4/1
  [VDDM_TailgaSWDFSRls_flg] -> Logical Operator32/1
  [VDDM_TailgaSWDet_flg] -> Logical Operator31/1
  Logical Operator29/1 -> DTC_Couter1/2
  [VDDM_TailgaSWCFSRls_flg] -> Logical Operator3/1
  SR_Latch2/1 -> Logical Operator28/2
  Constant60/1 -> DTC_Couter1/3
  Constant59/1 -> Logical Operator31/2
  Logical Operator32/1 -> SR_Latch2/2
  Constant56/1 -> Logical Operator29/2
  Relay1/1 -> SR_Latch2/1
  [DTC_clear_request] -> DTC_Info/4
  [VDDM_TailgaSWDet_flg] -> DTC_Info/1
  [VDDM_TailgaSWCFS_flg] -> DTC_Info/3
  [VDDM_TailgaSWPass_flg] -> DTC_Info/2
  DTC_Info/1 -> VDDM_TailgaSWDTC_raw32/1  "VDDM_TailgaSWDTC_raw32"
  Constant10/1 -> Switch11/3
  VPMM_PowerSta_enum/1 -> [VPMM_PowerSta_enum]
  VPMM_PwrStaSW_enum/1 -> [VPMM_PwrStaSW_enum]
  [VDDM_VCUTailgateSWSta_flg] -> VDDM_VCUTailgateSWSta_flg/1
  [VPMM_PowerSta_enum] -> Equal8/1
  Constant54/1 -> Switch15/1
  [DTC_clear_request] -> Logical Operator27/2
  Switch16/1 -> [VDDM_TailgaSWDFSRls_flg]
  Switch15/1 -> [VDDM_TailgaSWCFSRls_flg]  "VDDM_TailgaSWCFSRls_flg"
  Constant55/1 -> Switch15/3
  Constant45/1 -> Equal8/2
  Constant53/1 -> Switch16/3
  [VDDM_TailgaSWPass_flg] -> Switch16/2
  Equal8/1 -> Logical Operator27/1
  Constant52/1 -> Switch16/1
  Logical Operator27/1 -> Switch15/2
  Switch11/1 -> [VDDM_VCUTailgateSWSta_flg]  "VDDM_VCUTailgateSWSta_flg"
  Constant42/1 -> Switch11/1
  [VDDM_TailgaSWCFS_flg] -> Switch11/2
  task_time_s/1 -> [task_time_s]
  VINP_TailgaSW/1 -> [VINP_TailgaSWGPIO_flg]
  DTC_clear_request/1 -> [DTC_clear_request]
  Constant19/1 -> Equal3/2
  [VPMM_PwrStaSW_enum] -> Equal3/1
  SR_Latch3/1 -> [VDDM_TailgaSWPass_flg]  "VDDM_TailgaSWPass_flg"
  Equal1/1 -> Switch14/2
  Switch14/1 -> [VDDM_xxx_flg], Switch5/3
  Equal3/1 -> Switch10/2
  Unit Delay9/1 -> Data Type Conversion14/1
  Constant15/1 -> Timer1/4
  Timer/1 -> Relational Operator4/1, Unit Delay/1
  Constant16/1 -> Data Type Conversion7/1
  Timer1/1 -> Equal5/1
  Equal5/1 -> SR_Latch3/1
  Constant25/1 -> Test Detection Criteria2/3
  Constant18/1 -> Switch5/1
  [DTC_clear_request] -> Switch5/2
  [task_time_s] -> Test Detection Criteria2/2
  Relational Operator5/1 -> Unit Delay9/1, Equal4/2
  Logical Operator4/1 -> Timer/2
  Unit Delay/1 -> Subsystem/1
  Constant11/1 -> Timer/4
  [VINP_TailgaSWGPIO_flg] -> Relational Operator5/1
  Constant24/1 -> Equal5/2
  Constant17/1 -> Relational Operator4/2
  Logical Operator5/1 -> Subsystem/Trigger
  Constant23/1 -> Switch10/3
  SR_Latch1/1 -> Logical Operator5/1, Logical Operator4/1, Timer/1
  Data Type Conversion14/1 -> Equal4/1
  Constant22/1 -> Equal1/2
  Constant21/1 -> Switch14/3
  [task_time_s] -> Timer/3
  [task_time_s] -> Timer1/3
  Relational Operator4/1 -> Logical Operator6/2
  [VPMM_PwrStaSW_enum] -> Equal1/1
  Logical Operator6/1 -> [TailgaSWFault_flg], Switch14/1
  Switch10/1 -> Logical Operator7/1, Timer1/2
  Constant32/1 -> Relational Operator5/2
  [VDDM_xxx_flg] -> SR_Latch3/2
  Switch5/1 -> Data Type Conversion12/1
  Constant26/1 -> SR_Latch1/1
  Test Detection Criteria2/1 -> [VDDM_TailgaSWDet_flg]  "VDDM_TailgaSWDet_flg"
  Data Type Conversion7/1 -> Test Detection Criteria2/4
  [TailgaSWFault_flg] -> Switch10/1
  Logical Operator7/1 -> Timer1/1
  [VDDM_TailgaSWChange_flg] -> SR_Latch1/2
  Subsystem/1 -> Logical Operator6/1
  Data Type Conversion12/1 -> Test Detection Criteria2/1
  Equal4/1 -> [VDDM_TailgaSWChange_flg]

== system ddm/DDM/DDM/PMM/System conditions of ON to READY not satisfied/SR_Latch1 ==
  set : Inport
  reset : Inport  Port=2
  Logical Operator : Logic  AllPortsSameDT=off  OutDataTypeStr=boolean
  Logical Operator1 : Logic  Operator=NOT  AllPortsSameDT=off  OutDataTypeStr=boolean
  Switch1 : Switch  Criteria=u2 ~= 0  Threshold=0.5
      settings: AttributesFormatString=<Criteria=%<Criteria>>
  Switch2 : Switch  Criteria=u2 ~= 0  Threshold=0.5
      settings: AttributesFormatString=<Criteria=%<Criteria>>
  Unit Delay : UnitDelay  SampleTime=-1  HasFrameUpgradeWarning=on
  latched : Outport
  wires:
  Switch1/1 -> Unit Delay/1, latched/1
  set/1 -> Switch1/1, Logical Operator/1
  reset/1 -> Switch2/2, Logical Operator1/1
  Unit Delay/1 -> Switch2/3
  Switch2/1 -> Switch1/3
  Logical Operator/1 -> Switch1/2
  Logical Operator1/1 -> Logical Operator/2, Switch2/1

== system ddm/DDM/DDM/PMM/power up and power down/BMS HV relay closed fail ==
  note: Diagnostics and Fault Handling
  note: Fail Safe Operation After Failure Decision
  note: Fail Safe Operation During Failure Detection
  note: Release Condition During Failure Detection
  note: Test Pass Criteria
  note: Test Detection Criteria
  note: Release Condition After Failure Decision
  task_time_s : Inport
  VPMM_PowerSta_enum : Inport  Port=2
  VPMM_PwrStaSW_enum : Inport  Port=3
  VINP_HVBContactorSta_flg : Inport  Port=4
  VPMM_PowerUpFault_enum : Inport  Port=5
  DTC_clear_request : Inport  Port=6
  VPMM_PowerUpState_enum : Inport  Port=7
  Constant : Constant  Value=ENUM_PUFAULT_BATTUPFAIL
  Constant1 : Constant  Value=ENUM_PUSTATE_COMPLETED
  Constant10 : Constant  Value=KDDM_HVRlyCloDTC_cnt
  Constant11 : Constant  Value=KDDM_HVRlyCloPassSW_flg
  Constant15 : Constant  Value=KDDM_HVRlyCloCFSSW_flg
  Constant16 : Constant  Value=TRUE
  Constant19 : Constant  Value=ENUM_POWERSTA_OFF
  Constant{2,21,25,27} (4 alike) : Constant  Value=FALSE
  Constant20 : Constant  Value=KDDM_HVRlyCloDFSSW_flg
  Constant23 : Constant  Value=TRUE
  Constant24 : Constant  Value=TRUE
  Constant26 : Constant  Value=ENUM_PWRSTASW_OFF
  Constant38 : Constant  Commented=on  Value=KDDM_HVRlyCloDetTO_s
  Constant40 : Constant  Commented=on  Value=KDDM_HVRlyCloDTC_cnt
  Constant43 : Constant  Value=KDDM_HVRlyCloPassTO_s
  Constant44 : Constant  Value=KDDM_HVRlyCloDetSW_flg
  Constant8 : Constant  Value=KDDM_HVRlyCloPassTO_s
  DTC_Couter : hcu_lib/Basic_Blocks/DTC_Couter
  DTC_Info : hcu_lib/Basic_Blocks/DTC_Info
  Data Type Conversion1 : DataTypeConversion  OutDataTypeStr=uint8
  Equal : RelationalOperator  Operator=~=  OutDataTypeStr=boolean  RndMeth=Simplest
  Equal1 : RelationalOperator  Operator===  OutDataTypeStr=boolean  RndMeth=Simplest
  Equal2 : RelationalOperator  Operator===  OutDataTypeStr=boolean  RndMeth=Simplest
  Equal5 : RelationalOperator  OutDataTypeStr=boolean  RndMeth=Simplest
  Equal6 : RelationalOperator  Operator===  OutDataTypeStr=boolean  RndMeth=Simplest
  From48 : From  Commented=on  GotoTag=task_time_s
  Goto24 : Goto  Commented=on  GotoTag=VDDM_EDriveSysErrVCUErr_flg
  Logical Operator1 : Logic  Operator=NOT  AllPortsSameDT=off  OutDataTypeStr=boolean
  Logical Operator{5,12,15,18} (4 alike) : Logic  AllPortsSameDT=off  OutDataTypeStr=boolean
  Logical Operator19 : Logic  Inputs=3  AllPortsSameDT=off  OutDataTypeStr=boolean
  Logical Operator2 : Logic  Operator=OR  AllPortsSameDT=off  OutDataTypeStr=boolean
  Logical Operator3 : Logic  Operator=OR  Inputs=3  AllPortsSameDT=off  OutDataTypeStr=boolean
  Logical Operator4 : Logic  Operator=NOT  AllPortsSameDT=off  OutDataTypeStr=boolean
  Logical Operator6 : Logic  Operator=NOT  AllPortsSameDT=off  OutDataTypeStr=boolean
  Logical Operator7 : Logic  Operator=OR  AllPortsSameDT=off  OutDataTypeStr=boolean
  Logical Operator8 : Logic  Operator=OR  AllPortsSameDT=off  OutDataTypeStr=boolean
  Relay : Relay  OnSwitchValue=ONE_INT  OffSwitchValue=ZERO_INT
  SR_Latch1 : Subsystem  mask(SR_Latch){}
      mask help: SR latch function.
  SR_Latch3 : hcu_lib/Basic_Blocks/SR_Latch
  SR_Latch4 : hcu_lib/Basic_Blocks/SR_Latch
  Switch{,2,4..5} (4 alike) : Switch  Criteria=u2 ~= 0
  Test Detection Criteria : hcu_lib/Basic_Blocks/Test Detection Criteria  Commented=on
  Timer1 : hcu_lib/Basic_Blocks/Timer
  VDDM_HVRlyCloDTC_raw32 : Outport
  wires:
  Data Type Conversion1/1 -> [VDDM_HVRlyCloDTC_cnt]  "VDDM_HVRlyCloDTC_cnt"
  Logical Operator2/1 -> SR_Latch4/2
  Logical Operator7/1 -> SR_Latch3/2
  [DTC_clear_request] -> Logical Operator7/2
  [DTC_clear_request] -> Logical Operator2/2
  [VDDM_HVRlyCloCFS_flg] -> Logical Operator7/1
  [DTC_clear_request] -> Logical Operator1/1
  Constant44/1 -> Logical Operator19/2
  DTC_Couter/2 -> Data Type Conversion1/1
  Logical Operator15/1 -> DTC_Couter/2
  Relay/1 -> SR_Latch3/1
  [VDDM_HVRlyCloDet_flg] -> Logical Operator19/1
  Logical Operator1/1 -> Logical Operator19/3
  Logical Operator3/1 -> Logical Operator15/1
  [VDDM_HVRlyCloPass_flg] -> Logical Operator3/1
  Logical Operator12/1 -> [VDDM_HVRlyCloDFS_flg]  "VDDM_HVRlyCloDFS_flg"
  DTC_Couter/1 -> SR_Latch4/1
  Logical Operator19/1 -> DTC_Couter/1
  SR_Latch4/1 -> Logical Operator18/1
  Constant15/1 -> Logical Operator18/2
  [VDDM_HVRlyCloCFSRls_flg] -> Logical Operator2/1
  [VDDM_HVRlyCloCFSRls_flg] -> Logical Operator3/2
  [DTC_clear_request] -> Logical Operator3/3
  [VDDM_HVRlyCloDTC_cnt] -> Relay/1
  Constant10/1 -> DTC_Couter/3
  Logical Operator18/1 -> [VDDM_HVRlyCloCFS_flg]  "VDDM_HVRlyCloCFS_flg"
  Constant20/1 -> Logical Operator12/1
  Constant11/1 -> Logical Operator15/2
  SR_Latch3/1 -> Logical Operator12/2
  [VPMM_PowerUpState_enum] -> Equal2/1
  Constant1/1 -> Equal2/2
  Constant2/1 -> Switch2/1
  VPMM_PowerUpState_enum/1 -> [VPMM_PowerUpState_enum]
  [DTC_clear_request] -> DTC_Info/4
  Constant38/1 -> Test Detection Criteria/4
  [VDDM_HVRlyCloDet_flg] -> DTC_Info/1
  [VDDM_HVRlyCloCFS_flg] -> DTC_Info/3
  [VDDM_HVRlyCloPass_flg] -> DTC_Info/2
  DTC_Info/1 -> VDDM_HVRlyCloDTC_raw32/1  "VDDM_HVRlyCloDTC_raw32"
  Logical Operator5/1 -> [VDDM_HVRlyCloChk_flg]
  VPMM_PowerUpFault_enum/1 -> Equal1/1
  VINP_HVBContactorSta_flg/1 -> Logical Operator4/1
  Logical Operator4/1 -> Logical Operator5/1
  Equal1/1 -> Logical Operator5/2
  Constant/1 -> Equal1/2
  DTC_clear_request/1 -> [DTC_clear_request]
  Switch2/1 -> Logical Operator6/1, Timer1/2, SR_Latch1/2(reset)
  Timer1/1 -> Equal5/1
  [VDDM_HVRlyCloChk_flg] -> Switch5/1
  Constant19/1 -> Equal6/2
  Constant43/1 -> Timer1/4
  Constant27/1 -> Switch5/3
  Equal6/1 -> Logical Operator8/1
  SR_Latch1/1(latched) -> [VDDM_HVRlyCloPass_flg]  "VDDM_HVRlyCloPass_flg"
  Logical Operator6/1 -> Timer1/1
  Logical Operator8/1 -> Switch4/2
  Equal/1 -> Switch5/2
  Equal2/1 -> Switch2/2
  [DTC_clear_request] -> Logical Operator8/2
  [VDDM_HVRlyCloCFS_flg] -> Switch/2
  [VPMM_PwrStaSW_enum] -> Equal/1
  Constant25/1 -> Switch4/3
  Constant40/1 -> Test Detection Criteria/3
  Constant24/1 -> Switch4/1
  Switch5/1 -> [VDDM_HVRlyCloDet_flg]  "VDDM_HVRlyCloDet_flg"
  Switch/1 -> Goto24/1
  From48/1 -> Test Detection Criteria/2
  Constant26/1 -> Equal/2
  Constant16/1 -> Switch/1
  Constant23/1 -> Switch2/3
  [VPMM_PowerSta_enum] -> Equal6/1
  [task_time_s] -> Timer1/3
  Constant8/1 -> Equal5/2
  Switch4/1 -> [VDDM_HVRlyCloCFSRls_flg]  "VDDM_HVRlyCloCFSRls_flg"
  Equal5/1 -> SR_Latch1/1(set)
  Constant21/1 -> Switch/3
  VPMM_PowerSta_enum/1 -> [VPMM_PowerSta_enum]
  VPMM_PwrStaSW_enum/1 -> [VPMM_PwrStaSW_enum]
  task_time_s/1 -> [task_time_s]

== system ddm/DDM/DDM/PMM/power up and power down/BMS HV relay opened fail ==
  note: Diagnostics and Fault Handling
  note: Release Condition After Failure Decision
  note: Fail Safe Operation During Failure Detection
  note: Release Condition During Failure Detection
  note: Fail Safe Operation After Failure Decision
  note: Test Detection Criteria
  note: Test Pass Criteria
  task_time_s : Inport
  VPMM_PowerSta_enum : Inport  Port=2
  VPMM_PwrStaSW_enum : Inport  Port=3
  VPMM_PowerDownFault_enum : Inport  Port=4
  DTC_clear_request : Inport  Port=5
  VINP_HVBContactorSta_flg : Inport  Port=6
  Constant : Constant  Value=ENUM_PDFAULT_BATTPDFAIL
  Constant1 : Constant  Value=ENUM_PWRSTASW_OFF
  Constant10 : Constant  Value=KDDM_HVRlyOpDTC_cnt
  Constant11 : Constant  Value=KDDM_HVRlyOpPassSW_flg
  Constant15 : Constant  Value=KDDM_HVRlyOpCFSSW_flg
  Constant16 : Constant  Value=TRUE
  Constant17 : Constant  Value=KDDM_HVRlyOpPassTO_s
  Constant2 : Constant  Value=ZERO_INT
  Constant20 : Constant  Value=KDDM_HVRlyOpDFSSW_flg
  Constant21 : Constant  Value=FALSE
  Constant22 : Constant  Value=ENUM_PWRSTASW_OFF
  Constant23 : Constant  Value=TRUE
  Constant24 : Constant  Value=TRUE
  Constant25 : Constant  Value=FALSE
  Constant27 : Constant  Value=FALSE
  Constant38 : Constant  Commented=on  Value=KDDM_HVRlyOpDetTO_s
  Constant40 : Constant  Commented=on  Value=KDDM_HVRlyOpDTC_cnt
  Constant43 : Constant  Value=KDDM_HVRlyOpPassTO_s
  Constant44 : Constant  Value=KDDM_HVRlyOpDetSW_flg
  DTC_Couter : hcu_lib/Basic_Blocks/DTC_Couter
  DTC_Info : hcu_lib/Basic_Blocks/DTC_Info
  Data Type Conversion1 : DataTypeConversion  OutDataTypeStr=uint8
  Equal1 : RelationalOperator  Operator===  OutDataTypeStr=boolean  RndMeth=Simplest
  Equal2 : RelationalOperator  Operator=~=  OutDataTypeStr=boolean  RndMeth=Simplest
  Equal4 : RelationalOperator  Operator=~=  OutDataTypeStr=boolean  RndMeth=Simplest
  Equal6 : RelationalOperator  OutDataTypeStr=boolean  RndMeth=Simplest
  Equal7 : RelationalOperator  Operator===  OutDataTypeStr=boolean  RndMeth=Simplest
  From48 : From  Commented=on  GotoTag=task_time_s
  Logical Operator1 : Logic  Operator=NOT  AllPortsSameDT=off  OutDataTypeStr=boolean
  Logical Operator12 : Logic  AllPortsSameDT=off  OutDataTypeStr=boolean
  Logical Operator15 : Logic  AllPortsSameDT=off  OutDataTypeStr=boolean
  Logical Operator18 : Logic  AllPortsSameDT=off  OutDataTypeStr=boolean
  Logical Operator19 : Logic  Inputs=3  AllPortsSameDT=off  OutDataTypeStr=boolean
  Logical Operator2 : Logic  Operator=OR  AllPortsSameDT=off  OutDataTypeStr=boolean
  Logical Operator3 : Logic  Operator=OR  Inputs=3  AllPortsSameDT=off  OutDataTypeStr=boolean
  Logical Operator4 : Logic  Operator=OR  AllPortsSameDT=off  OutDataTypeStr=boolean
  Logical Operator6 : Logic  Operator=NOT  AllPortsSameDT=off  OutDataTypeStr=boolean
  Logical Operator8 : Logic  Operator=OR  AllPortsSameDT=off  OutDataTypeStr=boolean
  Relay : Relay  OnSwitchValue=ONE_INT  OffSwitchValue=ZERO_INT
  SR_Latch1 : Subsystem  mask(SR_Latch){}
      mask help: SR latch function.
  SR_Latch3 : hcu_lib/Basic_Blocks/SR_Latch
  SR_Latch4 : hcu_lib/Basic_Blocks/SR_Latch
  Switch{,1,4..5} (4 alike) : Switch  Criteria=u2 ~= 0
  Test Detection Criteria : hcu_lib/Basic_Blocks/Test Detection Criteria  Commented=on
  Timer1 : hcu_lib/Basic_Blocks/Timer
  VDDM_HVRlyOpDTC_raw32 : Outport
  VDDM_HVRlyOpFail_flg : Outport  Port=2
  VDDM_HVRlyOpCFS_flg : Outport  Port=3
  wires:
  [VDDM_HVRlyOpCFS_flg] -> VDDM_HVRlyOpCFS_flg/1
  Logical Operator18/1 -> [VDDM_HVRlyOpCFS_flg]  "VDDM_HVRlyOpCFS_flg"
  [VDDM_HVRlyOpPass_flg] -> Logical Operator3/1
  Data Type Conversion1/1 -> [VDDM_HVRlyOpDTC_cnt]  "VDDM_HVRlyOpDTC_cnt"
  [DTC_clear_request] -> Logical Operator1/1
  [DTC_clear_request] -> Logical Operator2/2
  [VDDM_HVRlyOpDet_flg] -> Logical Operator19/1
  Logical Operator3/1 -> Logical Operator15/1
  Relay/1 -> SR_Latch3/1
  Constant10/1 -> DTC_Couter/3
  SR_Latch4/1 -> Logical Operator18/1
  Logical Operator4/1 -> SR_Latch3/2
  Logical Operator15/1 -> DTC_Couter/2
  Constant20/1 -> Logical Operator12/1
  [VDDM_HVRlyOpDTC_cnt] -> Relay/1
  [VDDM_HVRlyOpCFSRls_flg] -> Logical Operator3/2
  Constant15/1 -> Logical Operator18/2
  Constant11/1 -> Logical Operator15/2
  DTC_Couter/1 -> SR_Latch4/1
  DTC_Couter/2 -> Data Type Conversion1/1
  Logical Operator19/1 -> DTC_Couter/1
  Constant44/1 -> Logical Operator19/2
  [VDDM_HVRlyOpCFS_flg] -> Logical Operator4/1
  [VDDM_HVRlyOpCFSRls_flg] -> Logical Operator2/1
  Logical Operator2/1 -> SR_Latch4/2
  SR_Latch3/1 -> Logical Operator12/2
  [DTC_clear_request] -> Logical Operator4/2
  [DTC_clear_request] -> Logical Operator3/3
  Logical Operator12/1 -> [VDDM_HVRlyOpDFS_flg]  "VDDM_HVRlyOpDFS_flg"
  Logical Operator1/1 -> Logical Operator19/3
  [DTC_clear_request] -> DTC_Info/4
  Constant38/1 -> Test Detection Criteria/4
  [VDDM_HVRlyOpDet_flg] -> DTC_Info/1
  [VDDM_HVRlyOpCFS_flg] -> DTC_Info/3
  [VDDM_HVRlyOpPass_flg] -> DTC_Info/2
  DTC_Info/1 -> VDDM_HVRlyOpDTC_raw32/1  "VDDM_HVRlyOpDTC_raw32"
  [VDDM_HVRlyOpFail_flg] -> VDDM_HVRlyOpFail_flg/1
  Equal1/1 -> [VDDM_HVRlyOpChk_flg]
  Constant/1 -> Equal1/2
  VPMM_PowerDownFault_enum/1 -> Equal1/1
  DTC_clear_request/1 -> [DTC_clear_request]
  [DTC_clear_request] -> Logical Operator8/2
  Constant16/1 -> Switch/1
  [VPMM_PwrStaSW_enum] -> Equal2/1
  Equal7/1 -> Logical Operator8/1
  Constant1/1 -> Equal2/2
  Switch5/1 -> [VDDM_HVRlyOpDet_flg]  "VDDM_HVRlyOpDet_flg"
  Constant40/1 -> Test Detection Criteria/3
  Logical Operator8/1 -> Switch4/2
  Logical Operator6/1 -> Timer1/1
  Switch/1 -> [VDDM_HVRlyOpFail_flg]  "VDDM_HVRlyOpFail_flg"
  From48/1 -> Test Detection Criteria/2
  Constant24/1 -> Switch4/1
  Equal6/1 -> SR_Latch1/1(set)
  Switch1/1 -> Timer1/2, SR_Latch1/2(reset), Logical Operator6/1
  Timer1/1 -> Equal6/1
  Constant25/1 -> Switch4/3
  Constant22/1 -> Equal4/2
  Constant43/1 -> Timer1/4
  [task_time_s] -> Timer1/3
  [VDDM_HVRlyOpChk_flg] -> Switch5/1
  Constant21/1 -> Switch/3
  Constant2/1 -> Equal7/2
  [VDDM_HVRlyOpCFS_flg] -> Switch/2
  [VDDM_HVRlyOpChk_flg] -> Switch1/1
  Switch4/1 -> [VDDM_HVRlyOpCFSRls_flg]  "VDDM_HVRlyOpCFSRls_flg"
  [VINP_HVBContactorSta_flg] -> Equal7/1
  [VPMM_PwrStaSW_enum] -> Equal4/1
  Constant27/1 -> Switch5/3
  Constant17/1 -> Equal6/2
  Constant23/1 -> Switch1/3
  Equal2/1 -> Switch1/2
  SR_Latch1/1(latched) -> [VDDM_HVRlyOpPass_flg]  "VDDM_HVRlyOpPass_flg"
  Equal4/1 -> Switch5/2
  VPMM_PowerSta_enum/1 -> [VPMM_PowerSta_enum]
  VPMM_PwrStaSW_enum/1 -> [VPMM_PwrStaSW_enum]
  task_time_s/1 -> [task_time_s]
  VINP_HVBContactorSta_flg/1 -> [VINP_HVBContactorSta_flg]
